simulink model "Test_Tricopter_Model"  (R2015a)
settings: Solver=ode3  SolverMode=SingleTasking  StartTime=0.0  StopTime=20  FixedStep=T_sim  RelTol=1e-3
PreLoadFcn:
  | LoadLibraries
values from neighbouring files (symbols this model uses):
  a = 10.26    [SetupComplete.m]
  A_x = 0.015    [SetupComplete.m]
  A_y = A_x    (= 0.015)    [SetupComplete.m]
  A_z = 0.16    [SetupComplete.m]
  C_d0 = 0.001193    [SetupComplete.m]
  C_x = 1.2    [SetupComplete.m]
  C_y = C_x    (= 1.2)    [SetupComplete.m]
  C_z = 2.2    [SetupComplete.m]
  CG_0 = [0,0,0.02]'    [SetupComplete.m]
  g = 9.81    [SetupComplete.m]
  h = 0.08    [SetupComplete.m]
  h_FA = 0.02    [SetupComplete.m]
  h_M = 0.064    [SetupComplete.m]
  I_BAC_0 = [ Ix,0,Ixz;0,Iy,0;Ixz,0,Iz]    [SetupComplete.m]
  I_prop = 1/4*M_eq*R^2*diag([1,1,2])    [SetupComplete.m]
  I_tube = [1/2*M_tube*R_tube_eq^2,0,  0  ;           0 ,1/3*M_tube*l_arm^2,0;             0  ,0,1/3*M_tube*l_arm^2]    [SetupComplete.m]
  Initial_Omegas = [1;1;1]*Omega_hover    [Run3Copter.m]
  J_FA = I_prop(1,1) + m_prop*h^2  + m_FA*h_FA^2 + m_M*h_M^2    [SetupComplete.m]
  J_T = J_m+1/2*M_eq*R^2    (= 2.000642e-05)    [SetupComplete.m]
  Ki = lqi(LM_4DOF_aug, Q,R)    [robust_controller.m]
  l = 0.3450    (= 0.345)    [NDI_components.m]    (also in SetupComplete.m; robust_controller.m)
  l_arm = 0.264    [SetupComplete.m]
  m = 3.51    [SetupComplete.m]
  m_0 = 2.61    [SetupComplete.m]
  m_FA = 0.02    [SetupComplete.m]
  m_M = 0.300    (= 0.3)    [SetupComplete.m]
  m_prop = 0.02    [SetupComplete.m]
  R = 0.1778    [SetupComplete.m]    (also in robust_controller.m = eye(4))
  rho = 1.15    [SetupComplete.m]
  sigma = b*c/(pi*R)    (= 0.107416159567)    [SetupComplete.m]
  T_sim = 0.01    [Run3Copter.m]
  theta_0 = 0.38397    [SetupComplete.m]
  theta_1 = -0.2967    [SetupComplete.m]
  trim_simplemodel = [0.589627915568 -2.20656039197 0 0.588313336084 0 0 0.588313330414 0 0]    [trimvalues.mat]
  V_4DOF_last = [0.0122475086001 0.00870447045314 -0.0292257707267 -0.0198753669721 -0.00290766514824 -0.0269511839788 0.0344308792695 -0.0305235710433 -0.0274078219028 -0.0329291952852 -0.0272335702183 -0.00643013158961 ... (1500 elements, 50x30)]    [NN_c_weights.mat]
  v_i0 = sqrt( 1/3*m*g/(2*rho*pi*R^2)  )    [SetupComplete.m]
  W_4DOF_last = [0.0132359246225 -0.0402459595001 -0.0221501781133 0.0046881519205 0.0457506835434 0.0464888535199 -0.0342386918322 0.0470592781761 0.0457166948243 -0.00146243512772 0.0300280468889 -0.0358113661373 ... (204 elements, 4x51)]    [NN_c_weights.mat]
undefined symbols (not defined in the file or in its folder): DOWN_0, EAST_0, Motor, NORTH_0, P_0, Prop, Q_0, R_0, sigmatest, U_0, V_0, v_i_adim, Vx_adim, Vz_adim, W_0
undefined symbols (not defined in the file): Initial_Torques, Rotation_sign, Tau_motors
libraries: simulink x61, XXCopter x32, vrlib x26, simulink_extras x6, aerolib6dofsys x3, qcatlib x3, dspinverses x3, lib_controller x2, aerolibtransform2 x2, aerolib6dof2 x1
(part 7 of 10)

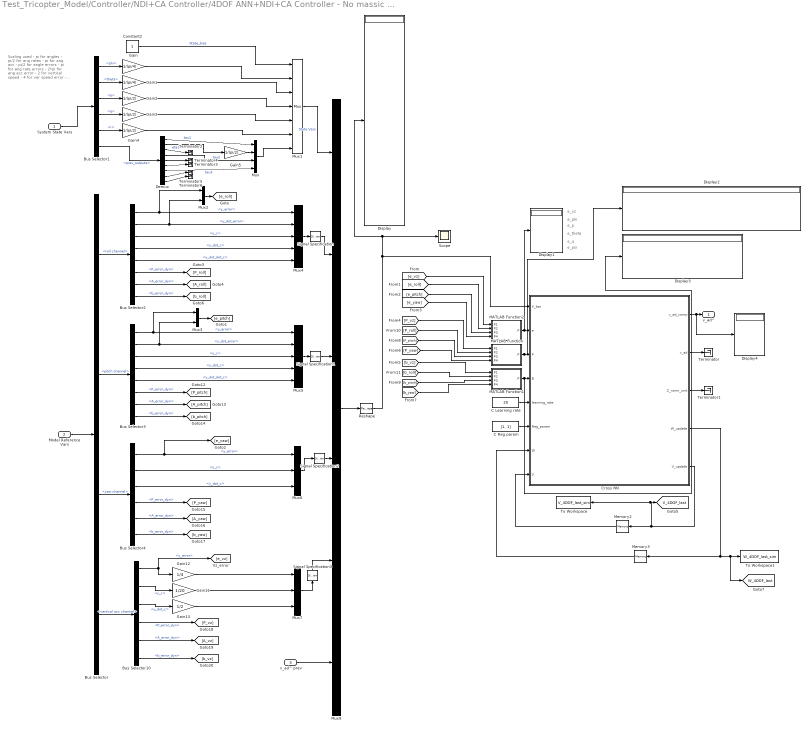
== system Test_Tricopter_Model/Controller/NDI+CA Controller/4DOF ANN+NDI+CA Controller - No massic update/Adaptive NN/Crossed NN ==
  note: e_vz
  note: Scaling used
      | - pi for angles
      | - pi/2 for ang rates
      | - pi for ang acc
      | - pi/2 for angle errors
      | - pi for ang rate errors
      | - 2*pi for ang acc error
      |
      | - 2 for vertical speed
      | - 4 for ver speed error
      | - 12 for vertical acc
      | - 18 for vertical acc error
  note: e_phi
  note: e_p
  note: e_theta
  note: e_q
  note: e_psi
  System State Vars : Inport
  Model Reference Vars : Inport  Port=2
  v_ad^ prev : Inport  Port=3
  Bus Selector : BusSelector  OutputSignals=roll channel,pitch channel,yaw channel,vertical acc channel
  Bus Selector1 : BusSelector  OutputSignals=phi,theta,p,q,r,prev_outputs
  Bus Selector10 : BusSelector  OutputSignals=y_error,y_c,y_dot_c,P_error_dyn,A_error_dyn,b_error_dyn
  Bus Selector2 : BusSelector  OutputSignals=y_error,y_dot_error,y_c,y_dot_c,y_dot_dot_c,P_error_dyn,A_error_dyn,b_error_dyn
  Bus Selector3 : BusSelector  OutputSignals=y_error,y_dot_error,y_c,y_dot_c,y_dot_dot_c,P_error_dyn,A_error_dyn,b_error_dyn
  Bus Selector4 : BusSelector  OutputSignals=y_error,y_c,y_dot_c,P_error_dyn,A_error_dyn,b_error_dyn
  C Learning rate : Constant  Value=20  SampleTime=T_sim
  C Reg param : Constant  Value=[1, 1]  SampleTime=T_sim
  Constant2 : Constant
  Cross NN : MATLAB Function  TreatAsAtomicUnit=on
  Demux : Demux  Outputs=9
  Display{,1..4} (5 alike) : Display
  Gain : Gain  Gain=1/(pi/4)
  Gain1 : Gain  Gain=1/(pi/4)
  Gain11 : Gain  Gain=1/20
  Gain12 : Gain  Gain=1/4
  Gain13 : Gain  Gain=1/2
  Gain{2..5} (4 alike) : Gain  Gain=1/(pi/2)
  MATLAB Function : MATLAB Function  TreatAsAtomicUnit=on
  MATLAB Function1 : MATLAB Function  TreatAsAtomicUnit=on
  MATLAB Function2 : MATLAB Function  TreatAsAtomicUnit=on
  Memory2 : Memory  X0=V_4DOF_last
  Memory3 : Memory  X0=W_4DOF_last
  Mux : Mux
  Mux1 : Mux  Inputs=7
  Mux2 : Mux  Inputs=2
  Mux3 : Mux  Inputs=2
  Mux4 : Mux  Inputs=5
  Mux5 : Mux  Inputs=5
  Mux6 : Mux  Inputs=3
  Mux7 : Mux  Inputs=3
  Mux9 : Mux  Inputs=6
  Reshape : Reshape
  Scope : Scope
      settings: SaveName=ScopeData8
  Signal Specification : SignalSpecification  Dimensions=5
  Signal Specification1 : SignalSpecification  Dimensions=5
  Signal Specification2 : SignalSpecification  Dimensions=3
  Signal Specification3 : SignalSpecification  Dimensions=3
  Terminator{,1..6} (7 alike) : Terminator
  To Workspace : ToWorkspace  VariableName=V_4DOF_last_sim  SampleTime=-1
      settings: MaxDataPoints=1  Save2DSignal=2-D array (concatenate along first dimension)
  To Workspace1 : ToWorkspace  VariableName=W_4DOF_last_sim  SampleTime=-1
      settings: MaxDataPoints=1  Save2DSignal=2-D array (concatenate along first dimension)
  v_ad^ : Outport
  tag scope: V_4DOF_last=global, W_4DOF_last=global
  wires:
  Cross NN/4(W_update) -> [W_4DOF_last], To Workspace1/1, Memory3/1
  Cross NN/5(V_update) -> Memory2/1, [V_4DOF_last], To Workspace/1
  Cross NN/2(v_ad) -> Terminator/1
  Memory3/1 -> Cross NN/7(W)
  Memory2/1 -> Cross NN/8(V)
  Cross NN/1(v_ad_comp) -> Display4/1, v_ad^/1
  C Learning rate/1 -> Cross NN/5(learning_rate)
  C Reg param/1 -> Cross NN/6(Reg_param)
  Cross NN/3(Z_norm_unit) -> Terminator1/1
  Mux9/1 -> Reshape/1
  Model Reference Vars/1 -> Bus Selector/1
  System State Vars/1 -> Bus Selector1/1
  Bus Selector1/1 -> Gain/1  "<phi>"
  Bus Selector1/2 -> Gain1/1  "<theta>"
  Bus Selector1/3 -> Gain2/1  "<p>"
  Bus Selector1/4 -> Gain3/1  "<q>"
  Bus Selector1/5 -> Gain4/1  "<r>"
  Bus Selector1/6 -> Demux/1  "<prev_outputs>"
  Gain5/1 -> Mux/2
  Mux1/1 -> Mux9/1  "State Vars"
  Mux/1 -> Mux1/7
  Gain2/1 -> Mux1/4
  Gain1/1 -> Mux1/3
  Gain3/1 -> Mux1/5
  Gain/1 -> Mux1/2
  Gain4/1 -> Mux1/6
  Constant2/1 -> Mux1/1  "State_bias"
  Bus Selector/1 -> Bus Selector2/1  "<roll channel>"
  Bus Selector2/1 -> Mux4/1, Mux2/1  "<y_error>"
  Bus Selector2/2 -> Mux4/2, Mux2/2  "<y_dot_error>"
  Bus Selector2/3 -> Mux4/3  "<y_c>"
  Bus Selector2/4 -> Mux4/4  "<y_dot_c>"
  Bus Selector2/5 -> Mux4/5  "<y_dot_dot_c>"
  Bus Selector/2 -> Bus Selector3/1  "<pitch channel>"
  Bus Selector3/1 -> Mux5/1, Mux3/1  "<y_error>"
  Bus Selector3/2 -> Mux5/2, Mux3/2  "<y_dot_error>"
  Bus Selector/3 -> Bus Selector4/1  "<yaw channel>"
  Bus Selector/4 -> Bus Selector10/1  "<vertical acc channel>"
  Bus Selector4/1 -> Mux6/1, [e_yaw]  "<y_error>"
  Mux2/1 -> [e_roll]
  Mux3/1 -> [e_pitch]
  Bus Selector2/6 -> [P_roll]  "<P_error_dyn>"
  Bus Selector2/7 -> [A_roll]  "<A_error_dyn>"
  Bus Selector2/8 -> [b_roll]  "<b_error_dyn>"
  Bus Selector10/1 -> Gain12/1, [e_vz]  "<y_error>"
  Bus Selector3/6 -> [P_pitch]  "<P_error_dyn>"
  Bus Selector3/7 -> [A_pitch]  "<A_error_dyn>"
  Bus Selector3/8 -> [b_pitch]  "<b_error_dyn>"
  Bus Selector4/4 -> [P_yaw]  "<P_error_dyn>"
  Bus Selector4/5 -> [A_yaw]  "<A_error_dyn>"
  Bus Selector4/6 -> [b_yaw]  "<b_error_dyn>"
  Bus Selector10/4 -> [P_vz]  "<P_error_dyn>"
  Bus Selector10/5 -> [A_vz]  "<A_error_dyn>"
  Bus Selector10/6 -> [b_vz]  "<b_error_dyn>"
  Bus Selector3/3 -> Mux5/3  "<y_c>"
  Bus Selector3/4 -> Mux5/4  "<y_dot_c>"
  Bus Selector3/5 -> Mux5/5  "<y_dot_dot_c>"
  Bus Selector4/2 -> Mux6/2  "<y_c>"
  Bus Selector4/3 -> Mux6/3  "<y_dot_c>"
  Bus Selector10/2 -> Gain11/1  "<y_c>"
  Bus Selector10/3 -> Gain13/1  "<y_dot_c>"
  v_ad^ prev/1 -> Mux9/6
  Reshape/1 -> Cross NN/1(X_bar), Display/1, Scope/1
  Mux5/1 -> Signal Specification1/1
  Gain12/1 -> Mux7/1
  Gain13/1 -> Mux7/3
  Gain11/1 -> Mux7/2
  Mux7/1 -> Signal Specification3/1
  MATLAB Function/1(P) -> Display2/1, Cross NN/3(P)
  [P_yaw] -> MATLAB Function/4(P4)
  [P_pitch] -> MATLAB Function/3(P3)
  [P_roll] -> MATLAB Function/2(P2)
  [P_vz] -> MATLAB Function/1(P1)
  MATLAB Function1/1(P) -> Display3/1, Cross NN/4(B)
  [b_vz] -> MATLAB Function1/1(P1)
  [b_roll] -> MATLAB Function1/2(P2)
  [b_pitch] -> MATLAB Function1/3(P3)
  [b_yaw] -> MATLAB Function1/4(P4)
  Demux/1 -> Mux/1  "tau1"
  Demux/2 -> Gain5/1  "eta1"
  Demux/4 -> Mux/3  "tau2"
  Demux/7 -> Mux/4  "tau3"
  Demux/3 -> Terminator2/1
  Demux/5 -> Terminator4/1
  Demux/6 -> Terminator3/1
  Demux/8 -> Terminator5/1
  Demux/9 -> Terminator6/1
  [e_yaw] -> MATLAB Function2/4(P4)
  [e_pitch] -> MATLAB Function2/3(P3)
  [e_roll] -> MATLAB Function2/2(P2)
  [e_vz] -> MATLAB Function2/1(P1)
  MATLAB Function2/1(P) -> Display1/1, Cross NN/2(e)
  Mux4/1 -> Signal Specification/1
  Signal Specification/1 -> Mux9/2
  Signal Specification1/1 -> Mux9/3
  Signal Specification2/1 -> Mux9/4
  Mux6/1 -> Signal Specification2/1
  Signal Specification3/1 -> Mux9/5

== system Test_Tricopter_Model/Controller/NDI+CA Controller/4DOF ANN+NDI+CA Controller - No massic update/Control Allocation 4DOF/Control Allocation 4DOF ==
  note: Position and rate limits for
      | tricopter actuators
  note: Weights used to normalize different
      | inputs between controllers.
      | Throttle - 0 to 1
      | Servo - 0 to 2*pi
  note: Enabler override saturations and override
      | them with zero to avoid actuators being
      | locked by control allocation algorithm
  Pseudocontrol input : Inport
  Effectiveness control matrix : Inport  Port=2
  "Control allocator Completed " : qcatlib/Control allocator Completed   alg=WLS  CA_type=QP  iter_max=10  gamma=1e6  k_B=4  m_B=4  T=0.01  tol=0
  Control positions deviation Weight W1 : Constant  Value=diag(1./[1,2*pi,1,1] )
  Control rate deviation Weight W2 : Constant  Value=diag(1./[1,2*pi,1,1] )
  Demux : Demux
  Enalbe/Disable : Constant
  Error Weight Wv2 : Constant  Value=blkdiag(1, 1/(2*pi), 1/(2*pi), 1/(2*pi))
  Ground{,1..4} (5 alike) : Ground
  Mux10 : Mux  Inputs=9
  Position limits 4 DOF : Constant  Value=[ [0,-deg2rad(165),0,0]', [1,deg2rad(160),1,1]']
  Rates limits 4DOF : Constant  Value=[ [-17,-1,-17,-17]', [17,1,17,17]']*1
  Reshape1 : Reshape  OutputDimensionality=Customize  OutputDimensions=[4,4]
  Reshape2 : Reshape  OutputDimensions=[6,1]
  Selector : Selector  InputPortWidth=9  Indices=[1 2 4 7]
  Terminator : Terminator
  Terminator1 : Terminator
  Unit Delay : UnitDelay  SampleTime=-1
  manual Initial saturations : Constant  Value=zeros(4,1)
  u desired : Constant  Value=zeros(4,1)
  Control output : Outport  PortDimensions=9
  wires:
  Pseudocontrol input/1 -> "Control allocator Completed "/1
  Unit Delay/1 -> "Control allocator Completed "/2
  "Control allocator Completed "/1 -> Unit Delay/1, Demux/1
  Ground4/1 -> Mux10/9
  Ground3/1 -> Mux10/8
  Ground2/1 -> Mux10/6
  Ground1/1 -> Mux10/5
  Ground/1 -> Mux10/3
  Demux/4 -> Mux10/7
  Demux/3 -> Mux10/4
  Demux/2 -> Mux10/2
  Demux/1 -> Mux10/1
  Mux10/1 -> Reshape2/1
  Reshape2/1 -> Control output/1
  Enalbe/Disable/1 -> "Control allocator Completed "/11
  manual Initial saturations/1 -> "Control allocator Completed "/10
  Control rate deviation Weight W2/1 -> "Control allocator Completed "/9
  Control positions deviation Weight W1/1 -> "Control allocator Completed "/8
  Error Weight Wv2/1 -> "Control allocator Completed "/7
  Rates limits 4DOF/1 -> "Control allocator Completed "/6
  Position limits 4 DOF/1 -> "Control allocator Completed "/5
  Reshape1/1 -> "Control allocator Completed "/4
  Effectiveness control matrix/1 -> Reshape1/1
  "Control allocator Completed "/3 -> Terminator1/1
  "Control allocator Completed "/2 -> Terminator/1
  [trimmed_input] -> Selector/1
  Selector/1 -> "Control allocator Completed "/3

== system Test_Tricopter_Model/Controller/NDI+CA Controller/4DOF ANN+NDI+CA Controller - No massic update/Control Allocation 4DOF/Pseudoinverse ==
  Pseudocontrol input : Inport
  Effectiveness control matrix : Inport  Port=2
  Demux : Demux
  Ground{,1..4} (5 alike) : Ground
  Mux10 : Mux  Inputs=9
  Product1 : Product  Multiplication=Matrix(*)
  Pseudoinverse : dspinverses/Pseudoinverse  wanterr=off
  Reshape1 : Reshape  OutputDimensions=[6,1]
  Control output : Outport  PortDimensions=9
  wires:
  Reshape1/1 -> Control output/1
  Pseudocontrol input/1 -> Product1/2
  Effectiveness control matrix/1 -> Pseudoinverse/1
  Pseudoinverse/1 -> Product1/1
  Mux10/1 -> Reshape1/1
  Demux/1 -> Mux10/1
  Demux/2 -> Mux10/2
  Demux/3 -> Mux10/4
  Demux/4 -> Mux10/7
  Ground/1 -> Mux10/3
  Ground1/1 -> Mux10/5
  Ground2/1 -> Mux10/6
  Ground3/1 -> Mux10/8
  Ground4/1 -> Mux10/9
  Product1/1 -> Demux/1

== system Test_Tricopter_Model/Controller/NDI+CA Controller/4DOF ANN+NDI+CA Controller - No massic update/Phi Model Reference/Reference Model1 ==
  u : Inport
  pch : Inport  Port=2
  Add : Sum  Inputs=|+-
  Add1 : Sum  Inputs=++-
  Integrator : Integrator
  Integrator1 : Integrator
  K_ref1 : Gain  Gain=2*xi*omega_n
  K_ref3 : Gain  Gain=omega_n^2
  y_dot_dot : Outport
  y_dot : Outport  Port=2
  y : Outport  Port=3
  wires:
  Integrator1/1 -> Integrator/1, K_ref1/1, y_dot/1
  Integrator/1 -> y/1, Add/2
  u/1 -> Add/1
  Add/1 -> K_ref3/1
  Add1/1 -> y_dot_dot/1, Integrator1/1  "y_dot_dot"
  K_ref3/1 -> Add1/2
  K_ref1/1 -> Add1/3
  pch/1 -> Add1/1

== system Test_Tricopter_Model/Controller/NDI+CA Controller/4DOF ANN+NDI+CA Controller - No massic update/Theta Model Reference1/Reference Model1 ==
  u : Inport
  pch : Inport  Port=2
  Add : Sum  Inputs=|+-
  Add1 : Sum  Inputs=++-
  Integrator : Integrator
  Integrator1 : Integrator
  K_ref1 : Gain  Gain=2*xi*omega_n
  K_ref3 : Gain  Gain=omega_n^2
  y_dot_dot : Outport
  y_dot : Outport  Port=2
  y : Outport  Port=3
  wires:
  Integrator1/1 -> Integrator/1, K_ref1/1, y_dot/1
  Integrator/1 -> y/1, Add/2
  u/1 -> Add/1
  Add/1 -> K_ref3/1
  Add1/1 -> y_dot_dot/1, Integrator1/1  "y_dot_dot"
  K_ref3/1 -> Add1/2
  K_ref1/1 -> Add1/3
  pch/1 -> Add1/1

== system Test_Tricopter_Model/Controller/NDI+CA Controller/4DOF NDI+CA Controller - No massic update/Control Allocation 4DOF/Control Allocation 4DOF ==
  note: Enabler override saturations and override
      | them with zero to avoid actuators being
      | locked by control allocation algorithm
  note: Weights used to normalize different
      | inputs between controllers.
      | Throttle - 0 to 1
      | Servo - 0 to 2*pi
  note: Position and rate limits for
      | tricopter actuators
  Pseudocontrol input : Inport
  Effectiveness control matrix : Inport  Port=2
  "Control allocator Completed " : qcatlib/Control allocator Completed   alg=WLS  CA_type=QP  iter_max=10  gamma=1e6  k_B=4  m_B=4  T=0.01  tol=0
  Control desired (0 to minimize control effort) : Constant  Value=zeros(1,4)
  Control positions deviation Weight W1 : Constant  Value=diag(1./[1,2*pi,1,1] )
  Control rate deviation Weight W2 : Constant  Value=diag(1./[1,2*pi,1,1] )
  Demux : Demux
  Enalbe/Disable : Constant
  Error Weight Wv2 : Constant  Value=blkdiag(1, 1/(2*pi), 1/(2*pi), 1/(2*pi))
  Ground{,1..4} (5 alike) : Ground
  Mux10 : Mux  Inputs=9
  Position limits 4 DOF : Constant  Value=[ [0,-deg2rad(165),0,0]', [1,deg2rad(160),1,1]']
  Rates limits 4DOF : Constant  Value=[ [-17,-1,-17,-17]', [17,1,17,17]']*1
  Reshape1 : Reshape  OutputDimensionality=Customize  OutputDimensions=[4,4]
  Reshape2 : Reshape  OutputDimensions=[6,1]
  Terminator : Terminator
  Terminator1 : Terminator
  Unit Delay : UnitDelay  SampleTime=-1
  manual Initial saturations : Constant  Value=zeros(4,1)
  Control output : Outport  PortDimensions=9
  wires:
  "Control allocator Completed "/2 -> Terminator/1
  "Control allocator Completed "/3 -> Terminator1/1
  Effectiveness control matrix/1 -> Reshape1/1
  Reshape1/1 -> "Control allocator Completed "/4
  Control desired (0 to minimize control effort)/1 -> "Control allocator Completed "/3
  Position limits 4 DOF/1 -> "Control allocator Completed "/5
  Rates limits 4DOF/1 -> "Control allocator Completed "/6
  Error Weight Wv2/1 -> "Control allocator Completed "/7
  Control positions deviation Weight W1/1 -> "Control allocator Completed "/8
  Control rate deviation Weight W2/1 -> "Control allocator Completed "/9
  manual Initial saturations/1 -> "Control allocator Completed "/10
  Enalbe/Disable/1 -> "Control allocator Completed "/11
  Reshape2/1 -> Control output/1
  Mux10/1 -> Reshape2/1
  Demux/1 -> Mux10/1
  Demux/2 -> Mux10/2
  Demux/3 -> Mux10/4
  Demux/4 -> Mux10/7
  Ground/1 -> Mux10/3
  Ground1/1 -> Mux10/5
  Ground2/1 -> Mux10/6
  Ground3/1 -> Mux10/8
  Ground4/1 -> Mux10/9
  "Control allocator Completed "/1 -> Demux/1, Unit Delay/1
  Unit Delay/1 -> "Control allocator Completed "/2
  Pseudocontrol input/1 -> "Control allocator Completed "/1

== system Test_Tricopter_Model/Controller/NDI+CA Controller/4DOF NDI+CA Controller - No massic update/Control Allocation 4DOF/Pseudoinverse ==
  Pseudocontrol input : Inport
  Effectiveness control matrix : Inport  Port=2
  Demux : Demux
  Ground{,1..4} (5 alike) : Ground
  Mux10 : Mux  Inputs=9
  Product1 : Product  Multiplication=Matrix(*)
  Pseudoinverse : dspinverses/Pseudoinverse  wanterr=off
  Reshape1 : Reshape  OutputDimensions=[6,1]
  Control output : Outport  PortDimensions=9
  wires:
  Product1/1 -> Demux/1
  Ground4/1 -> Mux10/9
  Ground3/1 -> Mux10/8
  Ground2/1 -> Mux10/6
  Ground1/1 -> Mux10/5
  Ground/1 -> Mux10/3
  Demux/4 -> Mux10/7
  Demux/3 -> Mux10/4
  Demux/2 -> Mux10/2
  Demux/1 -> Mux10/1
  Mux10/1 -> Reshape1/1
  Pseudoinverse/1 -> Product1/1
  Effectiveness control matrix/1 -> Pseudoinverse/1
  Pseudocontrol input/1 -> Product1/2
  Reshape1/1 -> Control output/1

== system Test_Tricopter_Model/3 Copter Complete/Arms Dynamics: Forces and Moments/4 DOF Arms Dynamics: Forces and Moments1/4 DOF Arms Dynamics: Forces and Moments1/Arm Dynamics/Aerodynamics Propeller ==
  note: Rotation_sign:
      |
      | * Anticlockwise from above rotation: Rotation_sign= -1
      | * Clockwise from above rotation: Rotation_sign= 1
  Omega : Inport
  h_ground : Inport  Port=2
  r_p : Inport  Port=3
  V^A : Inport  Port=4
  T_FaFb : Inport  Port=5
  2D vec norm : XXCopter/2D vec norm
  2D vec norm1 : XXCopter/2D vec norm
  Abs2 : Abs
  Add : Sum
  Aero Forces and Moments emb : Subsystem  AncestorBlock=XXCopter/Aero Forces and Moments emb  TreatAsAtomicUnit=on
  Dimensionless AB induced Vel Map : Lookup_n-D  BreakpointsForDimension1=Vx_adim  BreakpointsForDimension2=Vz_adim  BreakpointsForDimension3=[5, 7]  Table=v_i_adim  RndMeth=Simplest  InputSameDT=on
  Display : Display
  Divide : Product  Inputs=**
  F prop @ Fb : Product  Multiplication=Matrix(*)
  Gain : Gain  Gain=-1
  Gain1 : Gain  Gain=-1
  Induced hover Vel : Constant  Value=v_i0
  M prop @Fb : Product  Multiplication=Matrix(*)
  M_PAF : vrlib/Utilities/Cross Product
  Omega*R : Product  Inputs=**
  Prop Coefficients : MATLAB Function  TreatAsAtomicUnit=on
  Propeller Torque1 : Selector  IndexMode=Zero-based  InputPortWidth=3  Indices=2
  Radius Prop : Constant  Value=R
  Reaction! : Gain  Gain=-1
  Rotation_sign : Constant  Value=Rot_sign
  Scope : Scope
      settings: YMin=-20  YMax=2.5  SaveName=ScopeData9
  Sign : Signum
  V_A_x : Selector  InputPortWidth=3  Indices=[1 2]
  V_A_x,y : Selector  InputPortWidth=3  Indices=[1 2]
  V_A_x,y1 : Selector  InputPortWidth=3  Indices=[3]
  V_A_z : Selector  InputPortWidth=3  Indices=3
  Vx dimless : Product  Inputs=*/
  Vz dimless1 : Product  Inputs=*/
  lambda : Sum
  lambdaZ : Product  Inputs=*/
  lambda_i : Product  Inputs=*/
  mu : Product  Inputs=*/
  rho : Constant  Value=rho
  v_i dimension : Product  Inputs=**
  Prop_Torque_out : Outport
  Forces_prop @Fb : Outport  Port=2
  Moments_prop @Fb : Outport  Port=3
  wires:
  Abs2/1 -> Divide/1
  Sign/1 -> Divide/2
  Propeller Torque1/1 -> Abs2/1
  Divide/1 -> Prop_Torque_out/1
  rho/1 -> Aero Forces and Moments emb/7(rho)
  Reaction!/1 -> Aero Forces and Moments emb/9(Moment_sign)
  Prop Coefficients/4(C_Q) -> Aero Forces and Moments emb/4(C_Q), Sign/1
  mu/1 -> Prop Coefficients/2(mu)
  2D vec norm/1 -> Vx dimless/1
  M prop @Fb/1 -> Add/2
  M_PAF/1 -> Add/1
  r_p/1 -> M_PAF/1
  F prop @ Fb/1 -> Forces_prop @Fb/1, M_PAF/2
  Aero Forces and Moments emb/1(Fp) -> Display/1, Scope/1, F prop @ Fb/2
  T_FaFb/1 -> F prop @ Fb/1, M prop @Fb/1
  Rotation_sign/1 -> Reaction!/1
  h_ground/1 -> Aero Forces and Moments emb/8(h_ground)
  Add/1 -> Moments_prop @Fb/1
  Aero Forces and Moments emb/2("M_PM ") -> Propeller Torque1/1, M prop @Fb/2
  Omega/1 -> Omega*R/2, Aero Forces and Moments emb/5(Omega)
  V^A/1 -> V_A_z/1, V_A_x/1, V_A_x,y1/1, Aero Forces and Moments emb/6(V_A), V_A_x,y/1
  Prop Coefficients/3(C_MH) -> Aero Forces and Moments emb/3(C_MH)
  Prop Coefficients/2(C_H) -> Aero Forces and Moments emb/2(C_H)
  Prop Coefficients/1(C_T) -> Aero Forces and Moments emb/1(C_T)
  lambda/1 -> Prop Coefficients/1(lambda)
  Gain1/1 -> Vz dimless1/1
  lambdaZ/1 -> lambda/2
  lambda_i/1 -> lambda/1
  Gain/1 -> lambdaZ/1
  V_A_x,y1/1 -> Gain/1
  v_i dimension/1 -> lambda_i/1
  Dimensionless AB induced Vel Map/1 -> v_i dimension/1
  Induced hover Vel/1 -> Vx dimless/2, Vz dimless1/2, v_i dimension/2
  V_A_z/1 -> Gain1/1
  Vz dimless1/1 -> Dimensionless AB induced Vel Map/2
  V_A_x/1 -> 2D vec norm/1
  Vx dimless/1 -> Dimensionless AB induced Vel Map/1
  Omega*R/1 -> lambda_i/2, lambdaZ/2, mu/2
  2D vec norm1/1 -> mu/1
  V_A_x,y/1 -> 2D vec norm1/1
  Radius Prop/1 -> Omega*R/1

== system Test_Tricopter_Model/3 Copter Complete/Arms Dynamics: Forces and Moments/4 DOF Arms Dynamics: Forces and Moments1/4 DOF Arms Dynamics: Forces and Moments1/Arm Dynamics/Arms Kinematics ==
  Angles (rad) : Inport
  Angles_dot (rad/s) : Inport  Port=2
  Add : Sum
  Add3 : Sum
  Arm_no : Constant  Value=Arm_number
  Cross Product : vrlib/Utilities/Cross Product
  DCM Arm : MATLAB Function  TreatAsAtomicUnit=on
  Demux : Demux  Outputs=2
  Demux3 : Demux  Outputs=2
  Fa->Fb : Product  Multiplication=Matrix(*)
  Gain7 : Gain  Gain=[0;0;-1]
  Hub_position : Constant  Value=Arm_hub_position
  Matrix Multiply : Product  Multiplication=Matrix(*)
  Permute Dimensions : PermuteDimensions
  eta_dir : Gain  Gain=eta_dir
  gamma_dir : Gain  Gain=gamma_dir
  h arm : Constant  Value=h_prop
  r_p (m) : Outport
  r_p_dot (m/s) : Outport  Port=2
  T_F_a,Fb : Outport  Port=3
  omega_Ab (rad/s) : Outport  Port=4
  wires:
  Arm_no/1 -> DCM Arm/1(arm_no)
  Cross Product/1 -> r_p_dot (m/s)/1
  Fa->Fb/1 -> Add3/2, Cross Product/2
  Hub_position/1 -> Add3/1
  Gain7/1 -> Fa->Fb/2
  h arm/1 -> Gain7/1
  Add3/1 -> r_p (m)/1  "r_p (m)"
  Add/1 -> omega_Ab (rad/s)/1, Cross Product/1  "omega_Ab"
  eta_dir/1 -> Add/1
  Matrix Multiply/1 -> Add/2
  gamma_dir/1 -> Matrix Multiply/2
  Demux3/1 -> eta_dir/1  "eta_dot"
  Demux3/2 -> gamma_dir/1  "gamma_dot"
  Angles_dot (rad/s)/1 -> Demux3/1
  Demux/2 -> DCM Arm/3(gamma)
  Demux/1 -> DCM Arm/2(eta)
  Angles (rad)/1 -> Demux/1
  Permute Dimensions/1 -> Fa->Fb/1, Matrix Multiply/1, T_F_a,Fb/1  "T_F_a,Fb"
  DCM Arm/1(T_Fb_FA) -> Permute Dimensions/1

== system Test_Tricopter_Model/3 Copter Complete/Arms Dynamics: Forces and Moments/4 DOF Arms Dynamics: Forces and Moments1/4 DOF Arms Dynamics: Forces and Moments1/Arm Dynamics/Gyroscopic Moments ==
  T_FAFb : Inport
  omega_A  (rad/s) : Inport  Port=2
  omega_b  (rad/s) : Inport  Port=3
  Angles_dot (rad/s) : Inport  Port=4
  Angles_dot _dot(rad/s^2) : Inport  Port=5
  Omega (rad/s) : Inport  Port=6
  Omega_dot (rad/s^2) : Inport  Port=7
  Arm Inertia1 : MATLAB Function  TreatAsAtomicUnit=on
  Arm_axis : Constant  Value=Arm_axis
  Cross Product : vrlib/Utilities/Cross Product
  Cross Product1 : vrlib/Utilities/Cross Product
  Demux : Demux  Outputs=2
  Demux1 : Demux  Outputs=2
  Display : Display
  Display1 : Display
  Divide : Product  Inputs=**
  Divide1 : Product  Inputs=**
  F_A->F_b : Product  Multiplication=Matrix(*)
  F_A->F_b1 : Product  Multiplication=Matrix(*)
  Forearm Inertia : Constant  Value=J_FA
  Forearm Inertia1 : Constant  Value=J_FA
  Gain1 : Gain  Gain=[0;0;1]
  Gain3 : Gain  Gain=[0;0;1]
  L_FA : Product  Inputs=**
  L_eta_dot : Product  Multiplication=Matrix(*)
  L_prop : Product  Inputs=**
  Math Function{,2,4,6} (4 alike) : Math  Operator=square  SaturateOnIntegerOverflow=on
  Math Function{1,3,5,7} (4 alike) : Math  Operator=sqrt  SaturateOnIntegerOverflow=on
  Mux : Mux
  Propeller and motor inertia : Constant  Value=J_T
  Propeller and motor inertia1 : Constant  Value=J_T
  "Props, Motor and Forearm L @ F_A" : Sum
  "Props, Motor and Forearm dL/dt @ F_A" : Sum
  Rotation_sign : Constant  Value=Rot_sign
  Rotation_sign1 : Constant  Value=Rot_sign
  Sing of Gyro Moments : Gain  Gain=-1
  Sum of Elements{,1..3} (4 alike) : Sum  Inputs=+
  Total - Gyro Moment : Sum  Inputs=++++
  d L_FA/dt : Product  Inputs=**
  dL/dt of eta_dot_dot : Product  Multiplication=Matrix(*)
  dL/dt of prop : Product  Inputs=**
  eta_dir : Gain  Gain=eta_dir
  eta_dir1 : Gain  Gain=eta_dir
  gamma_dir : Gain  Gain=gamma_dir
  gamma_dir1 : Gain  Gain=gamma_dir
  M_gyro @Fb : Outport
  wires:
  Angles_dot (rad/s)/1 -> Demux/1
  Angles_dot _dot(rad/s^2)/1 -> Demux1/1
  Demux1/1 -> eta_dir/1  "eta_dot_dot_1"
  Arm Inertia1/1(J_Arm) -> Display/1, dL/dt of eta_dot_dot/1, L_eta_dot/1
  eta_dir/1 -> dL/dt of eta_dot_dot/2
  eta_dir1/1 -> L_eta_dot/2
  Demux/1 -> eta_dir1/1  "eta_dot_1"
  L_eta_dot/1 -> Cross Product/2
  omega_b  (rad/s)/1 -> Cross Product/1
  Demux1/2 -> gamma_dir/1  "gamma_dot_dot_1"
  gamma_dir/1 -> d L_FA/dt/1
  Forearm Inertia/1 -> d L_FA/dt/2
  Omega_dot (rad/s^2)/1 -> Gain3/1  "Omega_dot"
  Divide/1 -> dL/dt of prop/1
  Propeller and motor inertia/1 -> dL/dt of prop/2
  d L_FA/dt/1 -> "Props, Motor and Forearm dL/dt @ F_A"/1
  dL/dt of prop/1 -> "Props, Motor and Forearm dL/dt @ F_A"/2
  Demux/2 -> gamma_dir1/1  "gamma_dot"
  gamma_dir1/1 -> L_FA/1
  Forearm Inertia1/1 -> L_FA/2
  Divide1/1 -> L_prop/1
  Propeller and motor inertia1/1 -> L_prop/2
  L_FA/1 -> "Props, Motor and Forearm L @ F_A"/1
  L_prop/1 -> "Props, Motor and Forearm L @ F_A"/2
  Omega (rad/s)/1 -> Gain1/1  "Omega"
  "Props, Motor and Forearm dL/dt @ F_A"/1 -> F_A->F_b/2
  F_A->F_b/1 -> Math Function4/1, Total - Gyro Moment/2
  dL/dt of eta_dot_dot/1 -> Math Function6/1, Total - Gyro Moment/1
  Cross Product/1 -> Math Function2/1, Total - Gyro Moment/3
  "Props, Motor and Forearm L @ F_A"/1 -> F_A->F_b1/2
  T_FAFb/1 -> Arm Inertia1/1(T_FAFb), F_A->F_b/1, F_A->F_b1/1
  F_A->F_b1/1 -> Cross Product1/2
  omega_A  (rad/s)/1 -> Cross Product1/1
  Cross Product1/1 -> Math Function/1, Total - Gyro Moment/4
  Total - Gyro Moment/1 -> Sing of Gyro Moments/1
  Sing of Gyro Moments/1 -> M_gyro @Fb/1
  Arm_axis/1 -> Arm Inertia1/2(Arm_axis)
  Rotation_sign/1 -> Divide/1
  Gain3/1 -> Divide/2
  Rotation_sign1/1 -> Divide1/1
  Gain1/1 -> Divide1/2
  Mux/1 -> Display1/1
  Sum of Elements/1 -> Math Function1/1
  Math Function/1 -> Sum of Elements/1
  Sum of Elements1/1 -> Math Function3/1
  Math Function2/1 -> Sum of Elements1/1
  Sum of Elements2/1 -> Math Function5/1
  Math Function4/1 -> Sum of Elements2/1
  Sum of Elements3/1 -> Math Function7/1
  Math Function6/1 -> Sum of Elements3/1
  Math Function1/1 -> Mux/1
  Math Function3/1 -> Mux/2
  Math Function5/1 -> Mux/3
  Math Function7/1 -> Mux/4

== system Test_Tricopter_Model/3 Copter Complete/Arms Dynamics: Forces and Moments/4 DOF Arms Dynamics: Forces and Moments1/4 DOF Arms Dynamics: Forces and Moments1/Arm Dynamics/Servos Dynamics ==
  Com Angles (rad) : Inport
  Torques? : Inport  Port=2
  Add : Sum  Inputs=+-
  Add1 : Sum
  Demux : Demux  Outputs=2
  Derivative{,1..3} (4 alike) : Derivative  CoefficientInTFapproximation=derv_param
  Mux{,1..4} (5 alike) : Mux  Inputs=2
  Terminator : Terminator
  eta_1 : TransferFcn  Numerator=omega_n^2  Denominator=[1 xi*omega_n omega_n^2]
  gamma_1 : TransferFcn  Numerator=0  Denominator=1
  init_eta : Constant  Value=init_eta
  init_eta1 : Constant  Value=init_eta
  init_gamma : Constant  Value=init_gamma
  init_gamma1 : Constant  Value=init_gamma
  Angles Arms (rad) : Outport
  Angles_dot (rad/s) : Outport  Port=2
  Angles_dot_dot (rad/s^2) : Outport  Port=3
  wires:
  Add1/1 -> Angles Arms (rad)/1
  Mux4/1 -> Add1/1
  Mux/1 -> Add1/2
  init_gamma1/1 -> Mux4/2
  init_eta1/1 -> Mux4/1
  init_gamma/1 -> Mux3/2
  Mux3/1 -> Add/2
  init_eta/1 -> Mux3/1
  Add/1 -> Demux/1
  Torques?/1 -> Terminator/1
  Derivative/1 -> Derivative2/1, Mux1/1
  Derivative3/1 -> Mux2/2
  Derivative2/1 -> Mux2/1
  Derivative1/1 -> Mux1/2, Derivative3/1
  Mux2/1 -> Angles_dot_dot (rad/s^2)/1
  Mux1/1 -> Angles_dot (rad/s)/1
  gamma_1/1 -> Derivative1/1, Mux/2
  eta_1/1 -> Mux/1, Derivative/1
  Demux/2 -> gamma_1/1
  Demux/1 -> eta_1/1
  Com Angles (rad)/1 -> Add/1

== system Test_Tricopter_Model/3 Copter Complete/Arms Dynamics: Forces and Moments/4 DOF Arms Dynamics: Forces and Moments1/4 DOF Arms Dynamics: Forces and Moments1/Arm Dynamics1/Aerodynamics Propeller ==
  note: Rotation_sign:
      |
      | * Anticlockwise from above rotation: Rotation_sign= -1
      | * Clockwise from above rotation: Rotation_sign= 1
  Omega : Inport
  h_ground : Inport  Port=2
  r_p : Inport  Port=3
  V^A : Inport  Port=4
  T_FaFb : Inport  Port=5
  2D vec norm : XXCopter/2D vec norm
  2D vec norm1 : XXCopter/2D vec norm
  Abs2 : Abs
  Add : Sum
  Aero Forces and Moments emb : Subsystem  AncestorBlock=XXCopter/Aero Forces and Moments emb  TreatAsAtomicUnit=on
  Dimensionless AB induced Vel Map : Lookup_n-D  BreakpointsForDimension1=Vx_adim  BreakpointsForDimension2=Vz_adim  BreakpointsForDimension3=[5, 7]  Table=v_i_adim  RndMeth=Simplest  InputSameDT=on
  Divide : Product  Inputs=**
  F prop @ Fb : Product  Multiplication=Matrix(*)
  Gain : Gain  Gain=-1
  Gain1 : Gain  Gain=-1
  Induced hover Vel : Constant  Value=v_i0
  M prop @Fb : Product  Multiplication=Matrix(*)
  M_PAF : vrlib/Utilities/Cross Product
  Omega*R : Product  Inputs=**
  Prop Coefficients : MATLAB Function  TreatAsAtomicUnit=on
  Propeller Torque1 : Selector  IndexMode=Zero-based  InputPortWidth=3  Indices=2
  Radius Prop : Constant  Value=R
  Reaction! : Gain  Gain=-1
  Rotation_sign : Constant  Value=Rot_sign
  Sign : Signum
  V_A_x : Selector  InputPortWidth=3  Indices=[1 2]
  V_A_x,y : Selector  InputPortWidth=3  Indices=[1 2]
  V_A_x,y1 : Selector  InputPortWidth=3  Indices=[3]
  V_A_z : Selector  InputPortWidth=3  Indices=3
  Vx dimless : Product  Inputs=*/
  Vz dimless1 : Product  Inputs=*/
  lambda : Sum
  lambdaZ : Product  Inputs=*/
  lambda_i : Product  Inputs=*/
  mu : Product  Inputs=*/
  rho : Constant  Value=rho
  v_i dimension : Product  Inputs=**
  Prop_Torque_out : Outport
  Forces_prop @Fb : Outport  Port=2
  Moments_prop @Fb : Outport  Port=3
  wires:
  Abs2/1 -> Divide/1
  Sign/1 -> Divide/2
  Propeller Torque1/1 -> Abs2/1
  Divide/1 -> Prop_Torque_out/1
  rho/1 -> Aero Forces and Moments emb/7(rho)
  Reaction!/1 -> Aero Forces and Moments emb/9(Moment_sign)
  Prop Coefficients/4(C_Q) -> Aero Forces and Moments emb/4(C_Q), Sign/1
  mu/1 -> Prop Coefficients/2(mu)
  2D vec norm/1 -> Vx dimless/1
  M prop @Fb/1 -> Add/2
  M_PAF/1 -> Add/1
  r_p/1 -> M_PAF/1
  F prop @ Fb/1 -> Forces_prop @Fb/1, M_PAF/2
  Aero Forces and Moments emb/1(Fp) -> F prop @ Fb/2
  T_FaFb/1 -> F prop @ Fb/1, M prop @Fb/1
  Rotation_sign/1 -> Reaction!/1
  h_ground/1 -> Aero Forces and Moments emb/8(h_ground)
  Add/1 -> Moments_prop @Fb/1
  Aero Forces and Moments emb/2("M_PM ") -> Propeller Torque1/1, M prop @Fb/2
  Omega/1 -> Omega*R/2, Aero Forces and Moments emb/5(Omega)
  V^A/1 -> V_A_z/1, V_A_x/1, V_A_x,y1/1, Aero Forces and Moments emb/6(V_A), V_A_x,y/1
  Prop Coefficients/3(C_MH) -> Aero Forces and Moments emb/3(C_MH)
  Prop Coefficients/2(C_H) -> Aero Forces and Moments emb/2(C_H)
  Prop Coefficients/1(C_T) -> Aero Forces and Moments emb/1(C_T)
  lambda/1 -> Prop Coefficients/1(lambda)
  Gain1/1 -> Vz dimless1/1
  lambdaZ/1 -> lambda/2
  lambda_i/1 -> lambda/1
  Gain/1 -> lambdaZ/1
  V_A_x,y1/1 -> Gain/1
  v_i dimension/1 -> lambda_i/1
  Dimensionless AB induced Vel Map/1 -> v_i dimension/1
  Induced hover Vel/1 -> Vx dimless/2, Vz dimless1/2, v_i dimension/2
  V_A_z/1 -> Gain1/1
  Vz dimless1/1 -> Dimensionless AB induced Vel Map/2
  V_A_x/1 -> 2D vec norm/1
  Vx dimless/1 -> Dimensionless AB induced Vel Map/1
  Omega*R/1 -> lambda_i/2, lambdaZ/2, mu/2
  2D vec norm1/1 -> mu/1
  V_A_x,y/1 -> 2D vec norm1/1
  Radius Prop/1 -> Omega*R/1

== system Test_Tricopter_Model/3 Copter Complete/Arms Dynamics: Forces and Moments/4 DOF Arms Dynamics: Forces and Moments1/4 DOF Arms Dynamics: Forces and Moments1/Arm Dynamics1/Arms Kinematics ==
  Angles (rad) : Inport
  Angles_dot (rad/s) : Inport  Port=2
  Add : Sum
  Add3 : Sum
  Arm_no : Constant  Value=Arm_number
  Cross Product : vrlib/Utilities/Cross Product
  DCM Arm : MATLAB Function  TreatAsAtomicUnit=on
  Demux : Demux  Outputs=2
  Demux3 : Demux  Outputs=2
  Fa->Fb : Product  Multiplication=Matrix(*)
  Gain7 : Gain  Gain=[0;0;-1]
  Hub_position : Constant  Value=Arm_hub_position
  Matrix Multiply : Product  Multiplication=Matrix(*)
  Permute Dimensions : PermuteDimensions
  eta_dir : Gain  Gain=eta_dir
  gamma_dir : Gain  Gain=gamma_dir
  h arm : Constant  Value=h_prop
  r_p (m) : Outport
  r_p_dot (m/s) : Outport  Port=2
  T_F_a,Fb : Outport  Port=3
  omega_Ab (rad/s) : Outport  Port=4
  wires:
  Arm_no/1 -> DCM Arm/1(arm_no)
  Cross Product/1 -> r_p_dot (m/s)/1
  Fa->Fb/1 -> Add3/2, Cross Product/2
  Hub_position/1 -> Add3/1
  Gain7/1 -> Fa->Fb/2
  h arm/1 -> Gain7/1
  Add3/1 -> r_p (m)/1  "r_p (m)"
  Add/1 -> omega_Ab (rad/s)/1, Cross Product/1  "omega_Ab"
  eta_dir/1 -> Add/1
  Matrix Multiply/1 -> Add/2
  gamma_dir/1 -> Matrix Multiply/2
  Demux3/1 -> eta_dir/1  "eta_dot"
  Demux3/2 -> gamma_dir/1  "gamma_dot"
  Angles_dot (rad/s)/1 -> Demux3/1
  Demux/2 -> DCM Arm/3(gamma)
  Demux/1 -> DCM Arm/2(eta)
  Angles (rad)/1 -> Demux/1
  Permute Dimensions/1 -> Fa->Fb/1, Matrix Multiply/1, T_F_a,Fb/1  "T_F_a,Fb"
  DCM Arm/1(T_Fb_FA) -> Permute Dimensions/1

== system Test_Tricopter_Model/3 Copter Complete/Arms Dynamics: Forces and Moments/4 DOF Arms Dynamics: Forces and Moments1/4 DOF Arms Dynamics: Forces and Moments1/Arm Dynamics2/Aerodynamics Propeller ==
  note: Rotation_sign:
      |
      | * Anticlockwise from above rotation: Rotation_sign= -1
      | * Clockwise from above rotation: Rotation_sign= 1
  Omega : Inport
  h_ground : Inport  Port=2
  r_p : Inport  Port=3
  V^A : Inport  Port=4
  T_FaFb : Inport  Port=5
  2D vec norm : XXCopter/2D vec norm
  2D vec norm1 : XXCopter/2D vec norm
  Abs2 : Abs
  Add : Sum
  Aero Forces and Moments emb : Subsystem  AncestorBlock=XXCopter/Aero Forces and Moments emb  TreatAsAtomicUnit=on
  Dimensionless AB induced Vel Map : Lookup_n-D  BreakpointsForDimension1=Vx_adim  BreakpointsForDimension2=Vz_adim  BreakpointsForDimension3=[5, 7]  Table=v_i_adim  RndMeth=Simplest  InputSameDT=on
  Divide : Product  Inputs=**
  F prop @ Fb : Product  Multiplication=Matrix(*)
  Gain : Gain  Gain=-1
  Gain1 : Gain  Gain=-1
  Induced hover Vel : Constant  Value=v_i0
  M prop @Fb : Product  Multiplication=Matrix(*)
  M_PAF : vrlib/Utilities/Cross Product
  Omega*R : Product  Inputs=**
  Prop Coefficients : MATLAB Function  TreatAsAtomicUnit=on
  Propeller Torque1 : Selector  IndexMode=Zero-based  InputPortWidth=3  Indices=2
  Radius Prop : Constant  Value=R
  Reaction! : Gain  Gain=-1
  Rotation_sign : Constant  Value=Rot_sign
  Sign : Signum
  V_A_x : Selector  InputPortWidth=3  Indices=[1 2]
  V_A_x,y : Selector  InputPortWidth=3  Indices=[1 2]
  V_A_x,y1 : Selector  InputPortWidth=3  Indices=[3]
  V_A_z : Selector  InputPortWidth=3  Indices=3
  Vx dimless : Product  Inputs=*/
  Vz dimless1 : Product  Inputs=*/
  lambda : Sum
  lambdaZ : Product  Inputs=*/
  lambda_i : Product  Inputs=*/
  mu : Product  Inputs=*/
  rho : Constant  Value=rho
  v_i dimension : Product  Inputs=**
  Prop_Torque_out : Outport
  Forces_prop @Fb : Outport  Port=2
  Moments_prop @Fb : Outport  Port=3
  wires:
  Abs2/1 -> Divide/1
  Sign/1 -> Divide/2
  Propeller Torque1/1 -> Abs2/1
  Divide/1 -> Prop_Torque_out/1
  rho/1 -> Aero Forces and Moments emb/7(rho)
  Reaction!/1 -> Aero Forces and Moments emb/9(Moment_sign)
  Prop Coefficients/4(C_Q) -> Aero Forces and Moments emb/4(C_Q), Sign/1
  mu/1 -> Prop Coefficients/2(mu)
  2D vec norm/1 -> Vx dimless/1
  M prop @Fb/1 -> Add/2
  M_PAF/1 -> Add/1
  r_p/1 -> M_PAF/1
  F prop @ Fb/1 -> Forces_prop @Fb/1, M_PAF/2
  Aero Forces and Moments emb/1(Fp) -> F prop @ Fb/2
  T_FaFb/1 -> F prop @ Fb/1, M prop @Fb/1
  Rotation_sign/1 -> Reaction!/1
  h_ground/1 -> Aero Forces and Moments emb/8(h_ground)
  Add/1 -> Moments_prop @Fb/1
  Aero Forces and Moments emb/2("M_PM ") -> Propeller Torque1/1, M prop @Fb/2
  Omega/1 -> Omega*R/2, Aero Forces and Moments emb/5(Omega)
  V^A/1 -> V_A_z/1, V_A_x/1, V_A_x,y1/1, Aero Forces and Moments emb/6(V_A), V_A_x,y/1
  Prop Coefficients/3(C_MH) -> Aero Forces and Moments emb/3(C_MH)
  Prop Coefficients/2(C_H) -> Aero Forces and Moments emb/2(C_H)
  Prop Coefficients/1(C_T) -> Aero Forces and Moments emb/1(C_T)
  lambda/1 -> Prop Coefficients/1(lambda)
  Gain1/1 -> Vz dimless1/1
  lambdaZ/1 -> lambda/2
  lambda_i/1 -> lambda/1
  Gain/1 -> lambdaZ/1
  V_A_x,y1/1 -> Gain/1
  v_i dimension/1 -> lambda_i/1
  Dimensionless AB induced Vel Map/1 -> v_i dimension/1
  Induced hover Vel/1 -> Vx dimless/2, Vz dimless1/2, v_i dimension/2
  V_A_z/1 -> Gain1/1
  Vz dimless1/1 -> Dimensionless AB induced Vel Map/2
  V_A_x/1 -> 2D vec norm/1
  Vx dimless/1 -> Dimensionless AB induced Vel Map/1
  Omega*R/1 -> lambda_i/2, lambdaZ/2, mu/2
  2D vec norm1/1 -> mu/1
  V_A_x,y/1 -> 2D vec norm1/1
  Radius Prop/1 -> Omega*R/1

== system Test_Tricopter_Model/3 Copter Complete/Arms Dynamics: Forces and Moments/4 DOF Arms Dynamics: Forces and Moments1/4 DOF Arms Dynamics: Forces and Moments1/Arm Dynamics2/Arms Kinematics ==
  Angles (rad) : Inport
  Angles_dot (rad/s) : Inport  Port=2
  Add : Sum
  Add3 : Sum
  Arm_no : Constant  Value=Arm_number
  Cross Product : vrlib/Utilities/Cross Product
  DCM Arm : MATLAB Function  TreatAsAtomicUnit=on
  Demux : Demux  Outputs=2
  Demux3 : Demux  Outputs=2
  Fa->Fb : Product  Multiplication=Matrix(*)
  Gain7 : Gain  Gain=[0;0;-1]
  Hub_position : Constant  Value=Arm_hub_position
  Matrix Multiply : Product  Multiplication=Matrix(*)
  Permute Dimensions : PermuteDimensions
  eta_dir : Gain  Gain=eta_dir
  gamma_dir : Gain  Gain=gamma_dir
  h arm : Constant  Value=h_prop
  r_p (m) : Outport
  r_p_dot (m/s) : Outport  Port=2
  T_F_a,Fb : Outport  Port=3
  omega_Ab (rad/s) : Outport  Port=4
  wires:
  Arm_no/1 -> DCM Arm/1(arm_no)
  Cross Product/1 -> r_p_dot (m/s)/1
  Fa->Fb/1 -> Add3/2, Cross Product/2
  Hub_position/1 -> Add3/1
  Gain7/1 -> Fa->Fb/2
  h arm/1 -> Gain7/1
  Add3/1 -> r_p (m)/1  "r_p (m)"
  Add/1 -> omega_Ab (rad/s)/1, Cross Product/1  "omega_Ab"
  eta_dir/1 -> Add/1
  Matrix Multiply/1 -> Add/2
  gamma_dir/1 -> Matrix Multiply/2
  Demux3/1 -> eta_dir/1  "eta_dot"
  Demux3/2 -> gamma_dir/1  "gamma_dot"
  Angles_dot (rad/s)/1 -> Demux3/1
  Demux/2 -> DCM Arm/3(gamma)
  Demux/1 -> DCM Arm/2(eta)
  Angles (rad)/1 -> Demux/1
  Permute Dimensions/1 -> Fa->Fb/1, Matrix Multiply/1, T_F_a,Fb/1  "T_F_a,Fb"
  DCM Arm/1(T_Fb_FA) -> Permute Dimensions/1

== system Test_Tricopter_Model/3 Copter Complete/Arms Dynamics: Forces and Moments/4 DOF Arms Dynamics: Forces and Moments1/4 DOF Arms Dynamics: Forces and Moments1/Arm Dynamics2/Servos Dynamics ==
  Com Angles (rad) : Inport
  Torques? : Inport  Port=2
  Add : Sum  Inputs=+-
  Add1 : Sum
  Demux : Demux  Outputs=2
  Derivative{,1..3} (4 alike) : Derivative  CoefficientInTFapproximation=derv_param
  Mux{,1..4} (5 alike) : Mux  Inputs=2
  Terminator : Terminator
  eta_1 : TransferFcn  Numerator=0  Denominator=1
  eta_2 : TransferFcn  Numerator=0  Denominator=1
  init_eta : Constant  Value=init_eta
  init_eta1 : Constant  Value=init_eta
  init_gamma : Constant  Value=init_gamma
  init_gamma1 : Constant  Value=init_gamma
  Angles Arms (rad) : Outport
  Angles_dot (rad/s) : Outport  Port=2
  Angles_dot_dot (rad/s^2) : Outport  Port=3
  wires:
  Com Angles (rad)/1 -> Add/1
  Demux/1 -> eta_1/1
  Demux/2 -> eta_2/1
  eta_1/1 -> Derivative/1, Mux/1
  eta_2/1 -> Mux/2, Derivative1/1
  Mux1/1 -> Angles_dot (rad/s)/1
  Mux2/1 -> Angles_dot_dot (rad/s^2)/1
  Derivative1/1 -> Derivative3/1, Mux1/2
  Derivative2/1 -> Mux2/1
  Derivative3/1 -> Mux2/2
  Derivative/1 -> Mux1/1, Derivative2/1
  Torques?/1 -> Terminator/1
  Add/1 -> Demux/1
  init_eta/1 -> Mux3/1
  Mux3/1 -> Add/2
  init_gamma/1 -> Mux3/2
  init_eta1/1 -> Mux4/1
  init_gamma1/1 -> Mux4/2
  Mux/1 -> Add1/2
  Mux4/1 -> Add1/1
  Add1/1 -> Angles Arms (rad)/1

== system Test_Tricopter_Model/3 Copter Complete/Arms Dynamics: Forces and Moments/9 DOF Arms Dynamics: Forces and Moments/9 DOF Arms Dynamics: Forces and Moments/Arm Dynamics/Aerodynamics Propeller ==
  note: Rotation_sign:
      |
      | * Anticlockwise from above rotation: Rotation_sign= -1
      | * Clockwise from above rotation: Rotation_sign= 1
  Omega : Inport
  h_ground : Inport  Port=2
  r_p : Inport  Port=3
  V^A : Inport  Port=4
  T_FaFb : Inport  Port=5
  2D vec norm : XXCopter/2D vec norm
  2D vec norm1 : XXCopter/2D vec norm
  Abs2 : Abs
  Add : Sum
  Aero Forces and Moments emb : Subsystem  AncestorBlock=XXCopter/Aero Forces and Moments emb  TreatAsAtomicUnit=on
  Dimensionless AB induced Vel Map : Lookup_n-D  BreakpointsForDimension1=Vx_adim  BreakpointsForDimension2=Vz_adim  BreakpointsForDimension3=[5, 7]  Table=v_i_adim  RndMeth=Simplest  InputSameDT=on
  Divide : Product  Inputs=**
  F prop @ Fb : Product  Multiplication=Matrix(*)
  Gain : Gain  Gain=-1
  Gain1 : Gain  Gain=-1
  Induced hover Vel : Constant  Value=v_i0
  M prop @Fb : Product  Multiplication=Matrix(*)
  M_PAF : vrlib/Utilities/Cross Product
  Omega*R : Product  Inputs=**
  Prop Coefficients : MATLAB Function  TreatAsAtomicUnit=on
  Propeller Torque1 : Selector  IndexMode=Zero-based  InputPortWidth=3  Indices=2
  Radius Prop : Constant  Value=R
  Reaction! : Gain  Gain=-1
  Reaction!1 : Gain  Gain=sigmatest(1,2)
  Reaction!2 : Gain  Gain=sigmatest(1,3)
  Reaction!3 : Gain  Gain=sigmatest(1,4)
  Reaction!4 : Gain  Gain=sigmatest(1,1)
  Rotation_sign : Constant  Value=Rot_sign
  Sign : Signum
  V_A_x : Selector  InputPortWidth=3  Indices=[1 2]
  V_A_x,y : Selector  InputPortWidth=3  Indices=[1 2]
  V_A_x,y1 : Selector  InputPortWidth=3  Indices=[3]
  V_A_z : Selector  InputPortWidth=3  Indices=3
  Vx dimless : Product  Inputs=*/
  Vz dimless1 : Product  Inputs=*/
  lambda : Sum
  lambdaZ : Product  Inputs=*/
  lambda_i : Product  Inputs=*/
  mu : Product  Inputs=*/
  rho : Constant  Value=rho
  v_i dimension : Product  Inputs=**
  Prop_Torque_out : Outport
  Forces_prop @Fb : Outport  Port=2
  Moments_prop @Fb : Outport  Port=3
  wires:
  Abs2/1 -> Divide/1
  Sign/1 -> Divide/2
  Propeller Torque1/1 -> Abs2/1
  Divide/1 -> Prop_Torque_out/1
  rho/1 -> Aero Forces and Moments emb/7(rho)
  Reaction!/1 -> Aero Forces and Moments emb/9(Moment_sign)
  mu/1 -> Prop Coefficients/2(mu)
  2D vec norm/1 -> Vx dimless/1
  M prop @Fb/1 -> Add/2
  M_PAF/1 -> Add/1
  r_p/1 -> M_PAF/1
  F prop @ Fb/1 -> Forces_prop @Fb/1, M_PAF/2
  Aero Forces and Moments emb/1(Fp) -> F prop @ Fb/2
  T_FaFb/1 -> F prop @ Fb/1, M prop @Fb/1
  Rotation_sign/1 -> Reaction!/1
  h_ground/1 -> Aero Forces and Moments emb/8(h_ground)
  Add/1 -> Moments_prop @Fb/1
  Aero Forces and Moments emb/2("M_PM ") -> Propeller Torque1/1, M prop @Fb/2
  Omega/1 -> Omega*R/2, Aero Forces and Moments emb/5(Omega)
  V^A/1 -> V_A_z/1, V_A_x/1, V_A_x,y1/1, Aero Forces and Moments emb/6(V_A), V_A_x,y/1
  lambda/1 -> Prop Coefficients/1(lambda)
  Gain1/1 -> Vz dimless1/1
  lambdaZ/1 -> lambda/2
  lambda_i/1 -> lambda/1
  Gain/1 -> lambdaZ/1
  V_A_x,y1/1 -> Gain/1
  v_i dimension/1 -> lambda_i/1
  Dimensionless AB induced Vel Map/1 -> v_i dimension/1
  Induced hover Vel/1 -> Vx dimless/2, Vz dimless1/2, v_i dimension/2
  V_A_z/1 -> Gain1/1
  Vz dimless1/1 -> Dimensionless AB induced Vel Map/2
  V_A_x/1 -> 2D vec norm/1
  Vx dimless/1 -> Dimensionless AB induced Vel Map/1
  Omega*R/1 -> lambda_i/2, lambdaZ/2, mu/2
  2D vec norm1/1 -> mu/1
  V_A_x,y/1 -> 2D vec norm1/1
  Radius Prop/1 -> Omega*R/1
  Prop Coefficients/1(C_T) -> Reaction!4/1
  Prop Coefficients/2(C_H) -> Reaction!1/1
  Prop Coefficients/3(C_MH) -> Reaction!2/1
  Prop Coefficients/4(C_Q) -> Reaction!3/1
  Reaction!4/1 -> Aero Forces and Moments emb/1(C_T)
  Reaction!1/1 -> Aero Forces and Moments emb/2(C_H)
  Reaction!2/1 -> Aero Forces and Moments emb/3(C_MH)
  Reaction!3/1 -> Aero Forces and Moments emb/4(C_Q), Sign/1

== system Test_Tricopter_Model/3 Copter Complete/Arms Dynamics: Forces and Moments/9 DOF Arms Dynamics: Forces and Moments/9 DOF Arms Dynamics: Forces and Moments/Arm Dynamics/Arms Kinematics ==
  Angles (rad) : Inport
  Angles_dot (rad/s) : Inport  Port=2
  Add : Sum
  Add3 : Sum
  Arm_no : Constant  Value=Arm_number
  Cross Product : vrlib/Utilities/Cross Product
  DCM Arm : MATLAB Function  TreatAsAtomicUnit=on
  Demux : Demux  Outputs=2
  Demux3 : Demux  Outputs=2
  Fa->Fb : Product  Multiplication=Matrix(*)
  Gain7 : Gain  Gain=[0;0;-1]
  Hub_position : Constant  Value=Arm_hub_position
  Matrix Multiply : Product  Multiplication=Matrix(*)
  Permute Dimensions : PermuteDimensions
  eta_dir : Gain  Gain=eta_dir
  gamma_dir : Gain  Gain=gamma_dir
  h arm : Constant  Value=h_prop
  r_p (m) : Outport
  r_p_dot (m/s) : Outport  Port=2
  T_F_a,Fb : Outport  Port=3
  omega_Ab (rad/s) : Outport  Port=4
  wires:
  Arm_no/1 -> DCM Arm/1(arm_no)
  Cross Product/1 -> r_p_dot (m/s)/1
  Fa->Fb/1 -> Add3/2, Cross Product/2
  Hub_position/1 -> Add3/1
  Gain7/1 -> Fa->Fb/2
  h arm/1 -> Gain7/1
  Add3/1 -> r_p (m)/1  "r_p (m)"
  Add/1 -> omega_Ab (rad/s)/1, Cross Product/1  "omega_Ab"
  eta_dir/1 -> Add/1
  Matrix Multiply/1 -> Add/2
  gamma_dir/1 -> Matrix Multiply/2
  Demux3/1 -> eta_dir/1  "eta_dot"
  Demux3/2 -> gamma_dir/1  "gamma_dot"
  Angles_dot (rad/s)/1 -> Demux3/1
  Demux/2 -> DCM Arm/3(gamma)
  Demux/1 -> DCM Arm/2(eta)
  Angles (rad)/1 -> Demux/1
  Permute Dimensions/1 -> Fa->Fb/1, Matrix Multiply/1, T_F_a,Fb/1  "T_F_a,Fb"
  DCM Arm/1(T_Fb_FA) -> Permute Dimensions/1
